simulink model "Arduino_control_demonstration_day"  (R2025a)
settings: Solver=FixedStepDiscrete  StartTime=0.0  StopTime=inf  FixedStep=0.01  RelTol=1e-3  EnableMultiTasking=on
libraries: simulink x2, arduinolib x1
settings Model: SILPILModeSetting=veronly  ExtModeTrigDuration=2  Creator=Josh  LastModifiedBy=Josh
settings SolverCC: AutoInsertRateTranBlk=on
settings DataIOCC: Decimation=10
settings OptimizationCC: EnhancedBackFolding=on  PassReuseOutputArgsAs=Individual arguments  ZeroExternalMemoryAtStartup=off  ZeroInternalMemoryAtStartup=off  MaxStackSize=64  OptimizeBlockOrder=speed  DifferentSizesBufferReuse=on  OptimizationCustomize=off  EfficientTunableParamExpr=on
settings DebuggingCC: ParameterTunabilityLossMsg=error
settings HardwareCC: ProdBitPerInt=16.0  ProdBitPerPointer=16.0  ProdBitPerSizeT=16.0  ProdBitPerPtrDiffT=16.0  ProdLargestAtomicFloat=None  ProdWordSize=8.0  ProdHWDeviceType=Atmel->AVR  UseEmbeddedCoderFeatures=off  UseSimulinkCoderFeatures=off
settings SFSimCC: MATLABDynamicMemAlloc=off
settings RTWCC: SystemTargetFile=ert.tlc  HardwareBoard=Arduino Uno  TemplateMakefile=ert_default_tmf  Toolchain=Arduino AVR  BuildConfiguration=Faster Runs  Description=Embedded Coder
settings CodeAppCC: ForceParamTrailComments=on  IgnoreCustomStorageClasses=off  OperatorAnnotations=on  SimulinkDataObjDesc=on  SFDataObjDesc=on  MangleLength=10.0  InsertBlockDesc=on
settings ERTTargetCC: ExtModeTransport=3.0  ExtModeAutomaticAllocSize=off  ExtModeStaticAllocSize=250.0  InlinedParameterPlacement=Hierarchical  SupportContinuousTime=on  SupportNonInlinedSFcns=on  SupportVariableSizeSignals=on

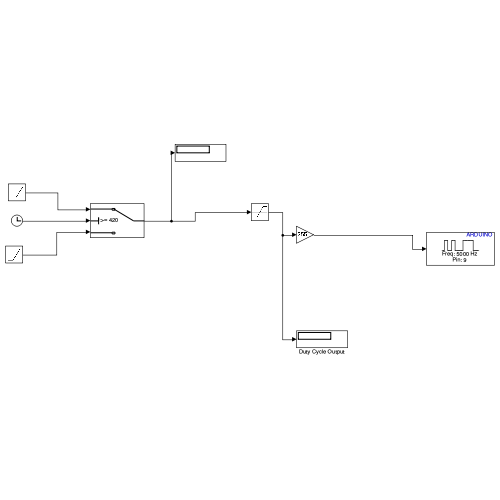
[thumbnail: Simulink's stored preview of the top-level diagram]
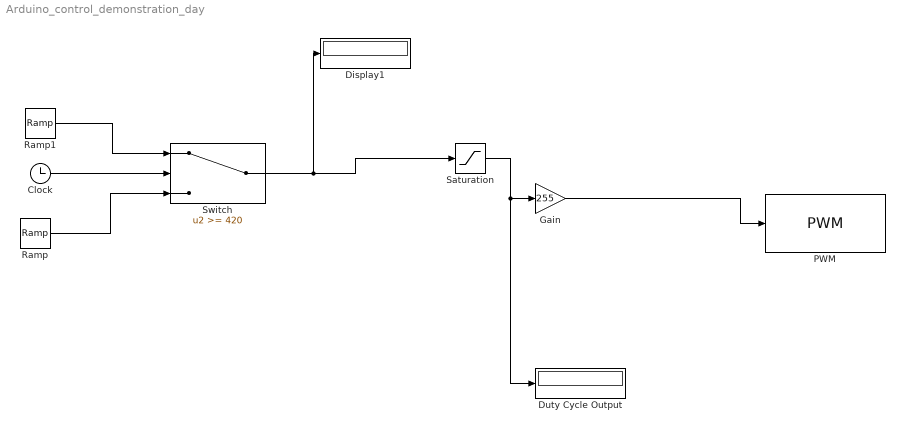
== system Arduino_control_demonstration_day ==
  Clock : Clock
  Display1 : Display
  Duty Cycle Output : Display
  Gain : Gain  Gain=255
  PWM : arduinolib/PWM  pinNumber=9  frequencyType=Specify  desiredFrequency=5000  achievableFrequency=5000
  Ramp : simulink/Sources/Ramp  slope=.7/6  start=0  InitialOutput=0
  Ramp1 : simulink/Sources/Ramp  slope=-.7/6  start=420  InitialOutput=0.7
  Saturation : Saturate  UpperLimit=0.7  LowerLimit=0
  Switch : Switch  Threshold=420  OutMax=0.7  SaturateOnIntegerOverflow=off  InputSameDT=off
  wires:
  Switch/1 -> Display1/1, Saturation/1
  Saturation/1 -> Duty Cycle Output/1, Gain/1
  Gain/1 -> PWM/1
  Clock/1 -> Switch/2
  Ramp1/1 -> Switch/1
  Ramp/1 -> Switch/3
